simulink model "saturated_systems_mitigation_example"  (R2021a)
settings: Solver=VariableStepAuto  StartTime=0.0  StopTime=simTime  RelTol=1e-3
values from neighbouring files (symbols this model uses):
  int_lim = int_limit(i)    [Anti_windup_example.m]
  K_a = K_A(i)    [Anti_windup_example.m]
  K_P = 1/abs(freqresp(G_ol,omega_c))    [Anti_windup_example.m]    (also in P_Lead_Lag.m = 1/abs(freqresp(G_ol,omega_c*1i)); Rate_limited_example.m; Rate_limited_exercise.m)
  step_size = 25    [Anti_windup_example.m]    (also in P_Lead_Lag.m = 1)
  tau_i = N_i/omega_c    [Anti_windup_example.m]    (also in P_Lead_Lag.m; Rate_limited_example.m = 0.75; Rate_limited_exercise.m = 0.666666666667)
undefined symbols (not defined in the file or in its folder): den_D, den_f, den_L, den_PI, num_D, num_f, num_L, num_PI
settings Model: Creator=dimpa  LastModifiedBy=dimpa
settings DataIOCC: Refine=154

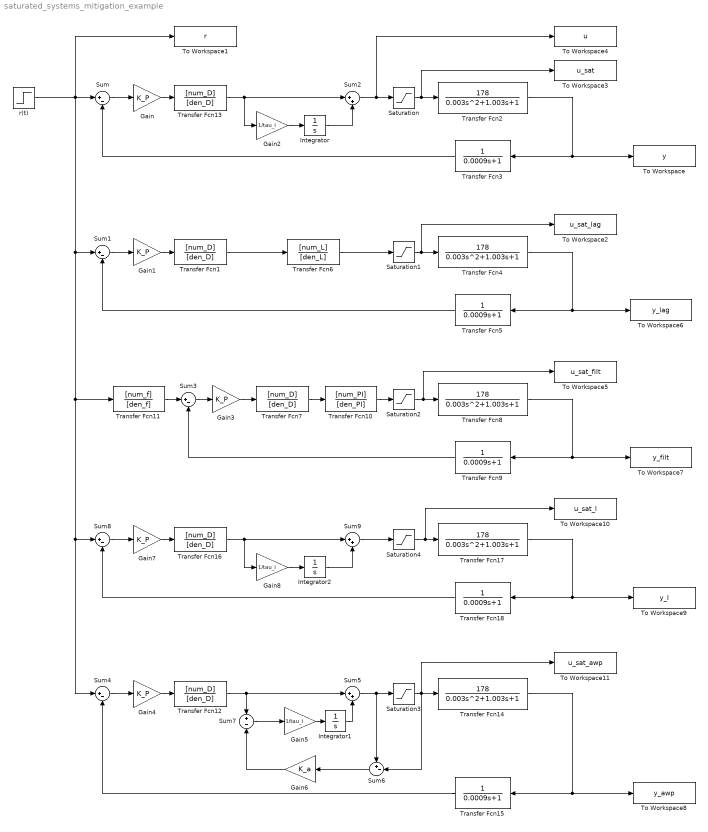
== system saturated_systems_mitigation_example ==
  Gain{,1,3..4,7} (5 alike) : Gain  Gain=K_P
  Gain2 : Gain  Gain=1/tau_i
  Gain5 : Gain  Gain=1/tau_i
  Gain6 : Gain  Gain=K_a
  Gain8 : Gain  Gain=1/tau_i
  Integrator : Integrator
  Integrator1 : Integrator
  Integrator2 : Integrator  LimitOutput=on  UpperSaturationLimit=int_lim  LowerSaturationLimit=-int_lim
  Saturation{,1..4} (5 alike) : Saturate  UpperLimit=4  LowerLimit=-4
  Sum{,1,3..4,8} (5 alike) : Sum  Inputs=|+-
  Sum2 : Sum  Inputs=|++
  Sum5 : Sum  Inputs=|++
  Sum6 : Sum  Inputs=+-|
  Sum7 : Sum  Inputs=+-
  Sum9 : Sum  Inputs=|++
  To Workspace : ToWorkspace  VariableName=y  SaveFormat=Timeseries  SampleTime=-1
  To Workspace1 : ToWorkspace  VariableName=r  SaveFormat=Timeseries  SampleTime=-1
  To Workspace10 : ToWorkspace  VariableName=u_sat_l  SaveFormat=Timeseries  SampleTime=-1
  To Workspace11 : ToWorkspace  VariableName=u_sat_awp  SaveFormat=Timeseries  SampleTime=-1
  To Workspace2 : ToWorkspace  VariableName=u_sat_lag  SaveFormat=Timeseries  SampleTime=-1
  To Workspace3 : ToWorkspace  VariableName=u_sat  SaveFormat=Timeseries  SampleTime=-1
  To Workspace4 : ToWorkspace  VariableName=u  SaveFormat=Timeseries  SampleTime=-1
  To Workspace5 : ToWorkspace  VariableName=u_sat_filt  SaveFormat=Timeseries  SampleTime=-1
  To Workspace6 : ToWorkspace  VariableName=y_lag  SaveFormat=Timeseries  SampleTime=-1
  To Workspace7 : ToWorkspace  VariableName=y_filt  SaveFormat=Timeseries  SampleTime=-1
  To Workspace8 : ToWorkspace  VariableName=y_awp  SaveFormat=Timeseries  SampleTime=-1
  To Workspace9 : ToWorkspace  VariableName=y_l  SaveFormat=Timeseries  SampleTime=-1
  Transfer Fcn{1,7,12..13,16} (5 alike) : TransferFcn  Numerator=[num_D]  Denominator=[den_D]
  Transfer Fcn10 : TransferFcn  Numerator=[num_PI]  Denominator=[den_PI]
  Transfer Fcn11 : TransferFcn  Numerator=[num_f]  Denominator=[den_f]
  Transfer Fcn{2,4,8,14,17} (5 alike) : TransferFcn  Numerator=[178]  Denominator=[0.003 1.003 1]
  Transfer Fcn{3,5,9,15,18} (5 alike) : TransferFcn  Denominator=[0.0009 1]
  Transfer Fcn6 : TransferFcn  Numerator=[num_L]  Denominator=[den_L]
  r(t) : Step  Time=0.1  After=step_size  SampleTime=0
  wires:
  Saturation/1 -> To Workspace3/1, Transfer Fcn2/1
  Transfer Fcn2/1 -> To Workspace/1, Transfer Fcn3/1
  Sum/1 -> Gain/1
  Gain/1 -> Transfer Fcn13/1
  Transfer Fcn3/1 -> Sum/2
  Sum2/1 -> Saturation/1, To Workspace4/1
  Transfer Fcn13/1 -> Gain2/1, Sum2/1
  Gain2/1 -> Integrator/1
  Integrator/1 -> Sum2/2
  Transfer Fcn1/1 -> Transfer Fcn6/1
  Transfer Fcn5/1 -> Sum1/2
  Gain1/1 -> Transfer Fcn1/1
  Sum1/1 -> Gain1/1
  Transfer Fcn4/1 -> To Workspace6/1, Transfer Fcn5/1
  Saturation1/1 -> To Workspace2/1, Transfer Fcn4/1
  Transfer Fcn6/1 -> Saturation1/1
  Transfer Fcn10/1 -> Saturation2/1
  Saturation2/1 -> To Workspace5/1, Transfer Fcn8/1
  Transfer Fcn8/1 -> Transfer Fcn9/1, To Workspace7/1
  Sum3/1 -> Gain3/1
  Gain3/1 -> Transfer Fcn7/1
  Transfer Fcn9/1 -> Sum3/2
  Transfer Fcn7/1 -> Transfer Fcn10/1
  Transfer Fcn11/1 -> Sum3/1
  Integrator1/1 -> Sum5/2
  Gain5/1 -> Integrator1/1
  Transfer Fcn12/1 -> Sum7/1, Sum5/1
  Sum5/1 -> Sum6/1, Saturation3/1
  Transfer Fcn15/1 -> Sum4/2
  Gain4/1 -> Transfer Fcn12/1
  Sum4/1 -> Gain4/1
  Transfer Fcn14/1 -> Transfer Fcn15/1, To Workspace8/1
  Saturation3/1 -> To Workspace11/1, Sum6/2, Transfer Fcn14/1
  Sum6/1 -> Gain6/1
  Sum7/1 -> Gain5/1
  Gain6/1 -> Sum7/2
  r(t)/1 -> Sum8/1, Sum4/1, Transfer Fcn11/1, Sum1/1, To Workspace1/1, Sum/1
  Integrator2/1 -> Sum9/2
  Gain8/1 -> Integrator2/1
  Transfer Fcn16/1 -> Sum9/1, Gain8/1
  Sum9/1 -> Saturation4/1
  Transfer Fcn18/1 -> Sum8/2
  Gain7/1 -> Transfer Fcn16/1
  Sum8/1 -> Gain7/1
  Transfer Fcn17/1 -> Transfer Fcn18/1, To Workspace9/1
  Saturation4/1 -> To Workspace10/1, Transfer Fcn17/1
